simulink model "Uppgift2"  (R2016a)
settings: Solver=VariableStepAuto  StartTime=0.0  StopTime=10.0  RelTol=1e-3
values from neighbouring files (symbols this model uses):
  C = A*8*eta*rKolv^2*L/rHole^4    (= 1.25663706144)    [Uppgift2script.m]
  K = 100    [Uppgift2script.m]
  M = 1    [Uppgift2script.m]
settings Model: Creator=Samuel  LastModifiedBy=Samuel

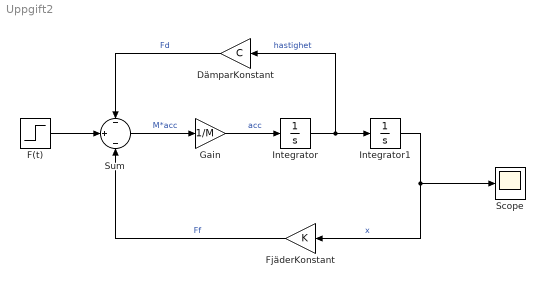
== system Uppgift2 ==
  DämparKonstant : Gain  Gain=C
  F(t) : Step  Time=0  SampleTime=0
  FjäderKonstant : Gain  Gain=K
  Gain : Gain  Gain=1/M
  Integrator : Integrator
  Integrator1 : Integrator
  Scope : Scope
  Sum : Sum  Inputs=-|+|-
  wires:
  F(t)/1 -> Sum/2
  Sum/1 -> Gain/1  "M*acc"
  Gain/1 -> Integrator/1  "acc"
  Integrator/1 -> DämparKonstant/1, Integrator1/1  "hastighet"
  Integrator1/1 -> Scope/1, FjäderKonstant/1  "x"
  FjäderKonstant/1 -> Sum/3  "Ff"
  DämparKonstant/1 -> Sum/1  "Fd"
